simulink model "ES2D7_Lift_Lab_2021"  (R2021a)
settings: Solver=VariableStepAuto  StartTime=0.0  StopTime=inf  RelTol=1e-3
settings Model: EnablePacing=on  PacingRate=1.100000  Creator=claire  LastModifiedBy=matteopenlington
settings SolverCC: AlgebraicLoopSolver=TrustRegion
settings DataIOCC: ReturnWorkspaceOutputs=off
settings DebuggingCC: SFMachineParentedDataDiag=warning  ArithmeticOperatorsInVariantConditions=warning
settings SFSimCC: CustomCodeUndefinedFunction=UseInterfaceOnly

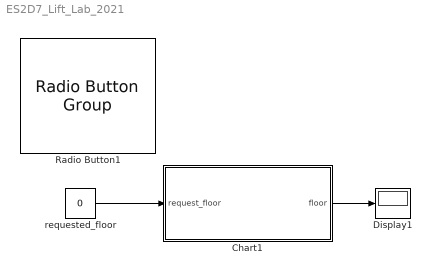
== system ES2D7_Lift_Lab_2021 ==
  Chart1 : Stateflow chart  TreatAsAtomicUnit=on
  Display1 : Display
  Radio Button1 : RadioButtonGroup  SelectedLabel=0  ButtonGroupName=Group
      settings: Values={{'0', '1', '2', '3', '4', '5'}, [0 1 2 3 4 5]}
  requested_floor : Constant  Value=0
  wires:
  requested_floor/1 -> Chart1/1(request_floor)
  Chart1/1(floor) -> Display1/1

== stateflow chart ES2D7_Lift_Lab_2021/Chart1 ==
  state Initial
    en:
    floor = 0;
  state idle
  state up
  state down
  up -> idle : after(2,sec){floor = floor+1}
  (default) -> Initial
  Initial -> idle
  idle -> up [order 1] : [request_floor>floor]
  idle -> down [order 2] : [request_floor<floor]
  down -> idle : after(2,sec){floor = floor -1}
  data: request_floor input; floor output
